simulink model "Model_10_1"  (R2021a)
settings: Solver=VariableStepAuto  StartTime=0.0  StopTime=10  RelTol=1e-3
InitFcn:
  | bx=25; %25
  | bl=50; %50
  | bc=0.1; %0.08
  | 
  | ml=2; %2
  | 
  | mc=0.5;
  | M2=0.5;
  | 
  | mt=5;
  | g=9.81;
  | l_ref=0.3; %0.3
  | l_ini=1;   %1
  | l=l_ini;
  | x_ref=1; %3
  | n1=1; %5
  | n2=1;
  | 
  | L_2=0;  %chieu dai day nang ha
  | 
  | theta1_ini=0*pi/180;
  | theta2_ini=0*pi/180;  %2*pi/180
  | 
  | L_tai=0.1;
  | %ADRC' s parameter caculation
  | %b0 = (1)/(mc+mt+ml);
  | b0=(ml+mc)/(mt*mc+2*ml*mc+mt*ml+ml^2+mc^2); %Enhanced-coupling
  | %k_ESO = 100;
  | k_ESO = 100;
  | T_set  = 3; %5;
  | 
  | s_cl = -5.85/T_set;
  | Kp   = s_cl^2;
  | Kd   = -2*s_cl;
  | 
  | s_ESO = k_ESO*s_cl;
  | l1        = -3*s_ESO;
  | l2        = 3*( s_ESO)^2;
  | l3        = -(s_ESO)^3;
  | 
  | %b1 = (mt+mc)/(mc*ml +mc*mt+ml*mt);
  | b1=1/(ml+mc);
  | k_ESO1 =100; %100
  | T_set1  = 3;   %3
  | s_cl1 = -5.85/T_set1;
  | Kp1   = s_cl1^2;
  | Kd1   = -2*s_cl1;
  | 
  | s_ESO1 = k_ESO1*s_cl1;
  | l11        = -3*s_ESO1;
  | l21        = 3*( s_ESO1)^2;
  | l31        = -(s_ESO1)^3;
  | 
  | 
  | %L1=l_ini;
  | L11=0.65;
  | L2=L_tai;
  | m1=2;
  | %m2=M2;
  | m=5;
  | ... (+35 lines)
libraries: neural x1372, simulink x44, simulink_extras x6
(part 44 of 58)

== matlab function Model_10_1/3_1_theta1 bang 0 n1=n2= 1/Ko co bx, bl, bc-1/Crane ==
  data: dx1 output; d1x input; l1 input; d1l1 input; the1 input; d1the1 input; the2 input; d1the2 input; Fx input; Fl input; dx2 output; dx3 output; dx4 output; dx5 output; dx6 output; m2 input; dx7 output; dx8 output; l2 input
function [dx1,dx2,dx3,dx4,dx5,dx6,dx7,dx8] = fcn(d1x,l1,d1l1,the1,d1the1,the2,d1the2,Fx,Fl,m2,l2)
 m =5; m1 =2; g =9.81;
 dx1=d1x;

 dx2 = (Fx*m2*cos(the1 - the2)^2 - Fx*m2 - Fx*m1 + Fx*m2*sin(the1 - the2)^2 + Fl*m1*sin(the1) + Fl*m2*sin(the1) - Fl*m2*sin(the1 - the2)*cos(the2) - d1the2^2*l2*m2^2*sin(the2) - g*m2^2*cos(the2)*sin(the2) - Fl*m2*cos(the1 - the2)^2*sin(the1) - g*m2^2*cos(the1 - the2)*sin(the1 - the2)*sin(the1)^2 + Fl*m2*cos(the1 - the2)*sin(the1 - the2)*cos(the1) + d1the2^2*l2*m2^2*cos(the1 - the2)*sin(the1) - d1the2^2*l2*m2^2*sin(the1 - the2)*cos(the1) - d1the2^2*l2*m1*m2*sin(the2) + g*m2^2*cos(the1 - the2)*cos(the1)*sin(the2) + g*m2^2*cos(the1 - the2)*cos(the2)*sin(the1) - g*m2^2*sin(the1 - the2)*cos(the1)*cos(the2) - g*m1*m2*cos(the2)*sin(the2) + g*m2^2*sin(the1 - the2)*sin(the1)*sin(the2) + d1the2^2*l2*m2^2*cos(the1 - the2)^2*sin(the2) - d1the2^2*l2*m2^2*cos(the1 - the2)^3*sin(the1) + d1the2^2*l2*m2^2*sin(the1 - the2)^3*cos(the1) - g*m2^2*cos(the1 - the2)^2*cos(the1)*sin(the1) + d1the2^2*l2*m2^2*sin(the1 - the2)^2*sin(the2) + g*m2^2*sin(the1 - the2)^2*cos(the1)*sin(the1) + g*m2^2*cos(the1 - the2)*sin(the1 - the2)*cos(the1)^2 - g*m1*m2*cos(the1 - the2)*sin(the1 - the2)*sin(the1)^2 + d1the2^2*l2*m1*m2*cos(the1 - the2)*sin(the1) - d1the2^2*l2*m1*m2*sin(the1 - the2)*cos(the1) + g*m1*m2*cos(the1 - the2)*cos(the1)*sin(the2) + g*m1*m2*cos(the1 - the2)*cos(the2)*sin(the1) - g*m1*m2*sin(the1 - the2)*cos(the1)*cos(the2) + g*m1*m2*sin(the1 - the2)*sin(the1)*sin(the2) + d1the2^2*l2*m2^2*cos(the1 - the2)^2*sin(the1 - the2)*cos(the1) - d1the2^2*l2*m2^2*cos(the1 - the2)*sin(the1 - the2)^2*sin(the1) - g*m1*m2*cos(the1 - the2)^2*cos(the1)*sin(the1) + g*m1*m2*sin(the1 - the2)^2*cos(the1)*sin(the1) + g*m1*m2*cos(the1 - the2)*sin(the1 - the2)*cos(the1)^2)/(m1^2*cos(the1)^2 - m*m2 - 2*m1*m2 - m*m1 + m2^2*cos(the1)^2 + m2^2*cos(the2)^2 + m1^2*sin(the1)^2 + m2^2*sin(the1)^2 + m2^2*cos(the1 - the2)^2 + m2^2*sin(the1 - the2)^2 - m1^2 - m2^2 + 2*m1*m2*cos(the1)^2 + m1*m2*cos(the2)^2 + 2*m1*m2*sin(the1)^2 + m*m2*cos(the1 - the2)^2 + m1*m2*cos(the1 - the2)^2 + m*m2*sin(the1 - the2)^2 + m1*m2*sin(the1 - the2)^2 - m2^2*cos(the1 - the2)^2*sin(the1)^2 - m2^2*sin(the1 - the2)^2*cos(the1)^2 - 2*m2^2*sin(the1 - the2)*cos(the2)*sin(the1) - 2*m2^2*cos(the1 - the2)*cos(the1)*cos(the2) - m1*m2*cos(the1 - the2)^2*sin(the1)^2 - m1*m2*sin(the1 - the2)^2*cos(the1)^2 + 2*m2^2*cos(the1 - the2)*sin(the1 - the2)*cos(the1)*sin(the1) - 2*m1*m2*sin(the1 - the2)*cos(the2)*sin(the1) - 2*m1*m2*cos(the1 - the2)*cos(the1)*cos(the2) + 2*m1*m2*cos(the1 - the2)*sin(the1 - the2)*cos(the1)*sin(the1));


 dx3=d1l1;

 dx4 = (Fx*m1^2*sin(the1) - Fl*m2^2 - Fl*m1^2 + Fx*m2^2*sin(the1) - d1the1^2*l1*m1^3 - d1the1^2*l1*m2^3 - g*m1^3*cos(the1) - g*m2^3*cos(the1) - Fl*m*m1 - Fl*m*m2 - 2*Fl*m1*m2 + Fl*m1^2*cos(the1)^2 + Fl*m2^2*cos(the1)^2 + Fl*m2^2*cos(the2)^2 + g*m1^3*cos(the1)^3 + g*m2^3*cos(the1)^3 + Fl*m2^2*cos(the1 - the2)^2 + 3*g*m1*m2^2*cos(the1)^3 + 3*g*m1^2*m2*cos(the1)^3 - Fx*m2^2*sin(the1 - the2)*cos(the2) - d1the2^2*l2*m2^3*cos(the1 - the2) + 2*Fx*m1*m2*sin(the1) + d1the1^2*l1*m1^3*cos(the1)^2 + d1the1^2*l1*m2^3*cos(the1)^2 + d1the1^2*l1*m2^3*cos(the2)^2 - g*m2^3*sin(the1 - the2)*sin(the2) + g*m2^3*cos(the1)*cos(the2)^2 + d1the1^2*l1*m1^3*sin(the1)^2 + d1the1^2*l1*m2^3*sin(the1)^2 + g*m1^3*cos(the1)*sin(the1)^2 + g*m2^3*cos(the1)*sin(the1)^2 + 2*Fl*m1*m2*cos(the1)^2 + Fl*m1*m2*cos(the2)^2 - Fx*m2^2*cos(the1 - the2)^2*sin(the1) + d1the1^2*l1*m2^3*cos(the1 - the2)^2 + d1the2^2*l2*m2^3*cos(the1 - the2)^3 - d1the1^2*l1*m*m1^2 - d1the1^2*l1*m*m2^2 - 3*d1the1^2*l1*m1*m2^2 - 3*d1the1^2*l1*m1^2*m2 + g*m2^3*cos(the1 - the2)^2*cos(the1) + d1the1^2*l1*m2^3*sin(the1 - the2)^2 - g*m*m1^2*cos(the1) - g*m*m2^2*cos(the1) - 3*g*m1*m2^2*cos(the1) - 3*g*m1^2*m2*cos(the1) + Fl*m*m2*cos(the1 - the2)^2 + Fl*m1*m2*cos(the1 - the2)^2 - g*m*m2^2*sin(the1 - the2)*sin(the2) - 2*g*m1*m2^2*sin(the1 - the2)*sin(the2) - g*m1^2*m2*sin(the1 - the2)*sin(the2) - d1the1^2*l1*m2^3*cos(the1 - the2)^2*sin(the1)^2 - d1the1^2*l1*m2^3*sin(the1 - the2)^2*cos(the1)^2 + 2*g*m1*m2^2*cos(the1)*cos(the2)^2 + g*m1^2*m2*cos(the1)*cos(the2)^2 + 3*d1the1^2*l1*m1*m2^2*sin(the1)^2 + 3*d1the1^2*l1*m1^2*m2*sin(the1)^2 + 3*g*m1*m2^2*cos(the1)*sin(the1)^2 + 3*g*m1^2*m2*cos(the1)*sin(the1)^2 + d1the2^2*l2*m2^3*sin(the1)*sin(the2) - 2*Fl*m2^2*cos(the1 - the2)*cos(the1)*cos(the2) + d1the1^2*l1*m*m2^2*cos(the1 - the2)^2 + 2*d1the1^2*l1*m1*m2^2*cos(the1 - the2)^2 + d1the1^2*l1*m1^2*m2*cos(the1 - the2)^2 + d1the2^2*l2*m*m2^2*cos(the1 - the2)^3 + d1the2^2*l2*m1*m2^2*cos(the1 - the2)^3 + g*m2^3*cos(the2)*sin(the1)*sin(the2) + g*m*m2^2*cos(the1 - the2)^2*cos(the1) + 2*g*m1*m2^2*cos(the1 - the2)^2*cos(the1) + g*m1^2*m2*cos(the1 - the2)^2*cos(the1) + d1the1^2*l1*m*m2^2*sin(the1 - the2)^2 + 2*d1the1^2*l1*m1*m2^2*sin(the1 - the2)^2 + d1the1^2*l1*m1^2*m2*sin(the1 - the2)^2 + Fx*m2^2*cos(the1 - the2)*sin(the1 - the2)*cos(the1) - Fx*m1*m2*sin(the1 - the2)*cos(the2) + d1the2^2*l2*m2^3*cos(the1 - the2)*cos(the1)^2 + d1the2^2*l2*m2^3*cos(the1 - the2)*cos(the2)^2 + g*m2^3*cos(the1 - the2)*sin(the1 - the2)*sin(the1) - 2*g*m2^3*cos(the1 - the2)*cos(the1)^2*cos(the2) - g*m2^3*cos(the1 - the2)*cos(the2)*sin(the1)^2 + g*m2^3*sin(the1 - the2)*cos(the1)^2*sin(the2) - Fx*m1*m2*cos(the1 - the2)^2*sin(the1) - d1the2^2*l2*m*m2^2*cos(the1 - the2) - 2*d1the2^2*l2*m1*m2^2*cos(the1 - the2) - d1the2^2*l2*m1^2*m2*cos(the1 - the2) - 2*d1the1^2*l1*m*m1*m2 + d1the2^2*l2*m2^3*cos(the1 - the2)*sin(the1 - the2)^2 - 2*g*m*m1*m2*cos(the1) + 3*d1the1^2*l1*m1*m2^2*cos(the1)^2 + 3*d1the1^2*l1*m1^2*m2*cos(the1)^2 + 2*d1the1^2*l1*m1*m2^2*cos(the2)^2 + d1the1^2*l1*m1^2*m2*cos(the2)^2 + 2*d1the2^2*l2*m1*m2^2*cos(the1 - the2)*cos(the1)^2 + d1the2^2*l2*m1^2*m2*cos(the1 - the2)*cos(the1)^2 + d1the2^2*l2*m1*m2^2*cos(the1 - the2)*cos(the2)^2 + g*m*m2^2*cos(the1 - the2)*sin(the1 - the2)*sin(the1) + 2*g*m1*m2^2*cos(the1 - the2)*sin(the1 - the2)*sin(the1) + g*m1^2*m2*cos(the1 - the2)*sin(the1 - the2)*sin(the1) - g*m*m1*m2*sin(the1 - the2)*sin(the2) - 2*d1the1^2*l1*m2^3*cos(the1 - the2)*cos(the1)*cos(the2) - 4*g*m1*m2^2*cos(the1 - the2)*cos(the1)^2*cos(the2) - 2*g*m1^2*m2*cos(the1 - the2)*cos(the1)^2*cos(the2) - 2*g*m1*m2^2*cos(the1 - the2)*cos(the2)*sin(the1)^2 - g*m1^2*m2*cos(the1 - the2)*cos(the2)*sin(the1)^2 - 2*d1the1^2*l1*m2^3*sin(the1 - the2)*cos(the2)*sin(the1) + d1the2^2*l2*m2^3*sin(the1 - the2)*cos(the1)*sin(the1) - d1the2^2*l2*m2^3*sin(the1 - the2)*cos(the2)*sin(the2) + 2*g*m1*m2^2*sin(the1 - the2)*cos(the1)^2*sin(the2) + g*m1^2*m2*sin(the1 - the2)*cos(the1)^2*sin(the2) - 2*Fl*m1*m2*cos(the1 - the2)*cos(the1)*cos(the2) + d1the1^2*l1*m*m1*m2*cos(the1 - the2)^2 - g*m2^3*cos(the1 - the2)*cos(the1)*sin(the1)*sin(the2) - g*m2^3*sin(the1 - the2)*cos(the1)*cos(the2)*sin(the1) + d1the2^2*l2*m*m2^2*cos(the1 - the2)*sin(the1 - the2)^2 + d1the2^2*l2*m1*m2^2*cos(the1 - the2)*sin(the1 - the2)^2 + g*m*m1*m2*cos(the1 - the2)^2*cos(the1) + d1the1^2*l1*m*m1*m2*sin(the1 - the2)^2 - 2*d1the2^2*l2*m2^3*cos(the1 - the2)^2*cos(the1)*cos(the2) - 2*d1the1^2*l1*m1*m2^2*cos(the1 - the2)^2*sin(the1)^2 - 2*d1the1^2*l1*m1*m2^2*sin(the1 - the2)^2*cos(the1)^2 - d1the1^2*l1*m1^2*m2*cos(the1 - the2)^2*sin(the1)^2 - d1the1^2*l1*m1^2*m2*sin(the1 - the2)^2*cos(the1)^2 + Fx*m1*m2*cos(the1 - the2)*sin(the1 - the2)*cos(the1) - d1the2^2*l2*m2^3*sin(the1 - the2)^2*cos(the1)*cos(the2) - d1the2^2*l2*m2^3*cos(the1 - the2)^2*sin(the1)*sin(the2) + 2*d1the2^2*l2*m1*m2^2*sin(the1)*sin(the2) + d1the2^2*l2*m1^2*m2*sin(the1)*sin(the2) + 2*g*m1*m2^2*cos(the2)*sin(the1)*sin(the2) + g*m1^2*m2*cos(the2)*sin(the1)*sin(the2) - d1the2^2*l2*m*m1*m2*cos(the1 - the2) - d1the2^2*l2*m1*m2^2*cos(the1 - the2)^2*sin(the1)*sin(the2) + g*m*m1*m2*cos(the1 - the2)*sin(the1 - the2)*sin(the1) + 2*d1the1^2*l1*m2^3*cos(the1 - the2)*sin(the1 - the2)*cos(the1)*sin(the1) + d1the2^2*l2*m2^3*cos(the1 - the2)*sin(the1 - the2)*cos(the1)*sin(the2) - d1the2^2*l2*m2^3*cos(the1 - the2)*sin(the1 - the2)*cos(the2)*sin(the1) - 4*d1the1^2*l1*m1*m2^2*cos(the1 - the2)*cos(the1)*cos(the2) - 2*d1the1^2*l1*m1^2*m2*cos(the1 - the2)*cos(the1)*cos(the2) - 4*d1the1^2*l1*m1*m2^2*sin(the1 - the2)*cos(the2)*sin(the1) - 2*d1the1^2*l1*m1^2*m2*sin(the1 - the2)*cos(the2)*sin(the1) + 2*d1the2^2*l2*m1*m2^2*sin(the1 - the2)*cos(the1)*sin(the1) + d1the2^2*l2*m1^2*m2*sin(the1 - the2)*cos(the1)*sin(the1) - d1the2^2*l2*m1*m2^2*sin(the1 - the2)*cos(the2)*sin(the2) - 2*g*m1*m2^2*cos(the1 - the2)*cos(the1)*sin(the1)*sin(the2) - 2*g*m1*m2^2*sin(the1 - the2)*cos(the1)*cos(the2)*sin(the1) - g*m1^2*m2*cos(the1 - the2)*cos(the1)*sin(the1)*sin(the2) - g*m1^2*m2*sin(the1 - the2)*cos(the1)*cos(the2)*sin(the1) - 2*d1the2^2*l2*m1*m2^2*cos(the1 - the2)^2*cos(the1)*cos(the2) - d1the2^2*l2*m1*m2^2*sin(the1 - the2)^2*cos(the1)*cos(the2) + 4*d1the1^2*l1*m1*m2^2*cos(the1 - the2)*sin(the1 - the2)*cos(the1)*sin(the1) + 2*d1the1^2*l1*m1^2*m2*cos(the1 - the2)*sin(the1 - the2)*cos(the1)*sin(the1) + d1the2^2*l2*m1*m2^2*cos(the1 - the2)*sin(the1 - the2)*cos(the1)*sin(the2) - d1the2^2*l2*m1*m2^2*cos(the1 - the2)*sin(the1 - the2)*cos(the2)*sin(the1))/((m1 + m2)*(m1^2*cos(the1)^2 - m*m2 - 2*m1*m2 - m*m1 + m2^2*cos(the1)^2 + m2^2*cos(the2)^2 + m1^2*sin(the1)^2 + m2^2*sin(the1)^2 + m2^2*cos(the1 - the2)^2 + m2^2*sin(the1 - the2)^2 - m1^2 - m2^2 + 2*m1*m2*cos(the1)^2 + m1*m2*cos(the2)^2 + 2*m1*m2*sin(the1)^2 + m*m2*cos(the1 - the2)^2 + m1*m2*cos(the1 - the2)^2 + m*m2*sin(the1 - the2)^2 + m1*m2*sin(the1 - the2)^2 - m2^2*cos(the1 - the2)^2*sin(the1)^2 - m2^2*sin(the1 - the2)^2*cos(the1)^2 - 2*m2^2*sin(the1 - the2)*cos(the2)*sin(the1) - 2*m2^2*cos(the1 - the2)*cos(the1)*cos(the2) - m1*m2*cos(the1 - the2)^2*sin(the1)^2 - m1*m2*sin(the1 - the2)^2*cos(the1)^2 + 2*m2^2*cos(the1 - the2)*sin(the1 - the2)*cos(the1)*sin(the1) - 2*m1*m2*sin(the1 - the2)*cos(the2)*sin(the1) - 2*m1*m2*cos(the1 - the2)*cos(the1)*cos(the2) + 2*m1*m2*cos(the1 - the2)*sin(the1 - the2)*cos(the1)*sin(the1)));


 dx5=d1the1;

 dx6 = -(g*m1^3*sin(the1)^3 - Fx*m2^2*cos(the1) - g*m1^3*sin(the1) - g*m2^3*sin(the1) - Fx*m1^2*cos(the1) + g*m2^3*sin(the1)^3 - 2*d1l1*d1the1*m1^3 - 2*d1l1*d1the1*m2^3 + 2*d1l1*d1the1*m1^3*cos(the1)^2 + 2*d1l1*d1the1*m2^3*cos(the1)^2 + 2*d1l1*d1the1*m2^3*cos(the2)^2 + Fl*m1^2*cos(the1)*sin(the1) + Fl*m2^2*cos(the1)*sin(the1) + 2*d1l1*d1the1*m1^3*sin(the1)^2 + 2*d1l1*d1the1*m2^3*sin(the1)^2 + 3*g*m1*m2^2*sin(the1)^3 + 3*g*m1^2*m2*sin(the1)^3 + Fx*m2^2*cos(the1 - the2)*cos(the2) - 2*Fx*m1*m2*cos(the1) + 2*d1l1*d1the1*m2^3*cos(the1 - the2)^2 - 2*d1l1*d1the1*m*m1^2 - 2*d1l1*d1the1*m*m2^2 - 6*d1l1*d1the1*m1*m2^2 - 6*d1l1*d1the1*m1^2*m2 + 2*d1l1*d1the1*m2^3*sin(the1 - the2)^2 - d1the2^2*l2*m2^3*sin(the1 - the2) + g*m2^3*cos(the1 - the2)*sin(the2) + Fl*m2^2*cos(the1 - the2)*sin(the1 - the2) + g*m1^3*cos(the1)^2*sin(the1) + g*m2^3*cos(the1)^2*sin(the1) + g*m2^3*cos(the2)^2*sin(the1) + Fx*m2^2*sin(the1 - the2)^2*cos(the1) + d1the2^2*l2*m2^3*sin(the1 - the2)^3 - g*m*m1^2*sin(the1) - g*m*m2^2*sin(the1) - 3*g*m1*m2^2*sin(the1) - 3*g*m1^2*m2*sin(the1) + g*m2^3*sin(the1 - the2)^2*sin(the1) - d1the2^2*l2*m2^3*cos(the1)*sin(the2) + 3*g*m1*m2^2*cos(the1)^2*sin(the1) + 3*g*m1^2*m2*cos(the1)^2*sin(the1) + 2*g*m1*m2^2*cos(the2)^2*sin(the1) + g*m1^2*m2*cos(the2)^2*sin(the1) - g*m2^3*cos(the1)*cos(the2)*sin(the2) - Fl*m2^2*cos(the1 - the2)*cos(the2)*sin(the1) - Fl*m2^2*sin(the1 - the2)*cos(the1)*cos(the2) + 2*Fl*m1*m2*cos(the1)*sin(the1) + d1the2^2*l2*m*m2^2*sin(the1 - the2)^3 + d1the2^2*l2*m1*m2^2*sin(the1 - the2)^3 + g*m*m2^2*sin(the1 - the2)^2*sin(the1) + 2*g*m1*m2^2*sin(the1 - the2)^2*sin(the1) + g*m1^2*m2*sin(the1 - the2)^2*sin(the1) + Fx*m1*m2*cos(the1 - the2)*cos(the2) - 4*d1l1*d1the1*m*m1*m2 - Fx*m2^2*cos(the1 - the2)*sin(the1 - the2)*sin(the1) + g*m2^3*cos(the1 - the2)*sin(the1 - the2)*cos(the1) + 6*d1l1*d1the1*m1*m2^2*cos(the1)^2 + 6*d1l1*d1the1*m1^2*m2*cos(the1)^2 + 4*d1l1*d1the1*m1*m2^2*cos(the2)^2 + 2*d1l1*d1the1*m1^2*m2*cos(the2)^2 - 2*d1l1*d1the1*m2^3*cos(the1 - the2)^2*sin(the1)^2 - 2*d1l1*d1the1*m2^3*sin(the1 - the2)^2*cos(the1)^2 + Fl*m*m2*cos(the1 - the2)*sin(the1 - the2) + Fl*m1*m2*cos(the1 - the2)*sin(the1 - the2) + 6*d1l1*d1the1*m1*m2^2*sin(the1)^2 + 6*d1l1*d1the1*m1^2*m2*sin(the1)^2 + d1the2^2*l2*m2^3*sin(the1 - the2)*cos(the2)^2 - g*m2^3*sin(the1 - the2)*cos(the1)^2*cos(the2) + d1the2^2*l2*m2^3*sin(the1 - the2)*sin(the1)^2 + 2*d1l1*d1the1*m*m2^2*cos(the1 - the2)^2 + 4*d1l1*d1the1*m1*m2^2*cos(the1 - the2)^2 + 2*d1l1*d1the1*m1^2*m2*cos(the1 - the2)^2 - g*m2^3*cos(the1 - the2)*sin(the1)^2*sin(the2) - 2*g*m2^3*sin(the1 - the2)*cos(the2)*sin(the1)^2 + Fx*m1*m2*sin(the1 - the2)^2*cos(the1) + 2*d1l1*d1the1*m*m2^2*sin(the1 - the2)^2 + 4*d1l1*d1the1*m1*m2^2*sin(the1 - the2)^2 + 2*d1l1*d1the1*m1^2*m2*sin(the1 - the2)^2 + d1the2^2*l2*m2^3*cos(the1 - the2)^2*sin(the1 - the2) - d1the2^2*l2*m*m2^2*sin(the1 - the2) - 2*d1the2^2*l2*m1*m2^2*sin(the1 - the2) - d1the2^2*l2*m1^2*m2*sin(the1 - the2) + g*m*m2^2*cos(the1 - the2)*sin(the2) + 2*g*m1*m2^2*cos(the1 - the2)*sin(the2) + g*m1^2*m2*cos(the1 - the2)*sin(the2) - 2*g*m*m1*m2*sin(the1) + g*m*m1*m2*cos(the1 - the2)*sin(the2) - 4*d1l1*d1the1*m1*m2^2*cos(the1 - the2)^2*sin(the1)^2 - 4*d1l1*d1the1*m1*m2^2*sin(the1 - the2)^2*cos(the1)^2 - 2*d1l1*d1the1*m1^2*m2*cos(the1 - the2)^2*sin(the1)^2 - 2*d1l1*d1the1*m1^2*m2*sin(the1 - the2)^2*cos(the1)^2 + d1the2^2*l2*m1*m2^2*sin(the1 - the2)*cos(the2)^2 + d1the2^2*l2*m2^3*cos(the1 - the2)*cos(the1)*sin(the1) + d1the2^2*l2*m2^3*cos(the1 - the2)*cos(the2)*sin(the2) - 2*g*m1*m2^2*sin(the1 - the2)*cos(the1)^2*cos(the2) - g*m1^2*m2*sin(the1 - the2)*cos(the1)^2*cos(the2) + 2*d1the2^2*l2*m1*m2^2*sin(the1 - the2)*sin(the1)^2 + d1the2^2*l2*m1^2*m2*sin(the1 - the2)*sin(the1)^2 - g*m2^3*cos(the1 - the2)*cos(the1)*cos(the2)*sin(the1) - 2*g*m1*m2^2*cos(the1 - the2)*sin(the1)^2*sin(the2) - 4*g*m1*m2^2*sin(the1 - the2)*cos(the2)*sin(the1)^2 - g*m1^2*m2*cos(the1 - the2)*sin(the1)^2*sin(the2) - 2*g*m1^2*m2*sin(the1 - the2)*cos(the2)*sin(the1)^2 - Fl*m1*m2*cos(the1 - the2)*cos(the2)*sin(the1) - Fl*m1*m2*sin(the1 - the2)*cos(the1)*cos(the2) + d1the2^2*l2*m*m2^2*cos(the1 - the2)^2*sin(the1 - the2) + d1the2^2*l2*m1*m2^2*cos(the1 - the2)^2*sin(the1 - the2) + g*m2^3*sin(the1 - the2)*cos(the1)*sin(the1)*sin(the2) + g*m*m1*m2*sin(the1 - the2)^2*sin(the1) - d1the2^2*l2*m2^3*cos(the1 - the2)^2*cos(the2)*sin(the1) - 2*d1the2^2*l2*m1*m2^2*cos(the1)*sin(the2) - d1the2^2*l2*m1^2*m2*cos(the1)*sin(the2) - Fx*m1*m2*cos(the1 - the2)*sin(the1 - the2)*sin(the1) + d1the2^2*l2*m2^3*sin(the1 - the2)^2*cos(the1)*sin(the2) - 2*d1the2^2*l2*m2^3*sin(the1 - the2)^2*cos(the2)*sin(the1) - 2*g*m1*m2^2*cos(the1)*cos(the2)*sin(the2) - g*m1^2*m2*cos(the1)*cos(the2)*sin(the2) - 4*d1l1*d1the1*m2^3*cos(the1 - the2)*cos(the1)*cos(the2) - 4*d1l1*d1the1*m2^3*sin(the1 - the2)*cos(the2)*sin(the1) + 2*d1l1*d1the1*m*m1*m2*cos(the1 - the2)^2 + 2*d1l1*d1the1*m*m1*m2*sin(the1 - the2)^2 - d1the2^2*l2*m*m1*m2*sin(the1 - the2) + g*m*m2^2*cos(the1 - the2)*sin(the1 - the2)*cos(the1) + 2*g*m1*m2^2*cos(the1 - the2)*sin(the1 - the2)*cos(the1) + g*m1^2*m2*cos(the1 - the2)*sin(the1 - the2)*cos(the1) + d1the2^2*l2*m1*m2^2*sin(the1 - the2)^2*cos(the1)*sin(the2) - 2*d1the2^2*l2*m1*m2^2*sin(the1 - the2)^2*cos(the2)*sin(the1) + g*m*m1*m2*cos(the1 - the2)*sin(the1 - the2)*cos(the1) - 8*d1l1*d1the1*m1*m2^2*cos(the1 - the2)*cos(the1)*cos(the2) - 4*d1l1*d1the1*m1^2*m2*cos(the1 - the2)*cos(the1)*cos(the2) - d1the2^2*l2*m2^3*cos(the1 - the2)*sin(the1 - the2)*cos(the1)*cos(the2) - 8*d1l1*d1the1*m1*m2^2*sin(the1 - the2)*cos(the2)*sin(the1) - 4*d1l1*d1the1*m1^2*m2*sin(the1 - the2)*cos(the2)*sin(the1) - d1the2^2*l2*m2^3*cos(the1 - the2)*sin(the1 - the2)*sin(the1)*sin(the2) + 2*d1the2^2*l2*m1*m2^2*cos(the1 - the2)*cos(the1)*sin(the1) + d1the2^2*l2*m1^2*m2*cos(the1 - the2)*cos(the1)*sin(the1) + d1the2^2*l2*m1*m2^2*cos(the1 - the2)*cos(the2)*sin(the2) - 2*g*m1*m2^2*cos(the1 - the2)*cos(the1)*cos(the2)*sin(the1) - g*m1^2*m2*cos(the1 - the2)*cos(the1)*cos(the2)*sin(the1) + 2*g*m1*m2^2*sin(the1 - the2)*cos(the1)*sin(the1)*sin(the2) + g*m1^2*m2*sin(the1 - the2)*cos(the1)*sin(the1)*sin(the2) + 4*d1l1*d1the1*m2^3*cos(the1 - the2)*sin(the1 - the2)*cos(the1)*sin(the1) - d1the2^2*l2*m1*m2^2*cos(the1 - the2)^2*cos(the2)*sin(the1) + 8*d1l1*d1the1*m1*m2^2*cos(the1 - the2)*sin(the1 - the2)*cos(the1)*sin(the1) + 4*d1l1*d1the1*m1^2*m2*cos(the1 - the2)*sin(the1 - the2)*cos(the1)*sin(the1) - d1the2^2*l2*m1*m2^2*cos(the1 - the2)*sin(the1 - the2)*cos(the1)*cos(the2) - d1the2^2*l2*m1*m2^2*cos(the1 - the2)*sin(the1 - the2)*sin(the1)*sin(the2))/(l1*(m1 + m2)*(m1^2*cos(the1)^2 - m*m2 - 2*m1*m2 - m*m1 + m2^2*cos(the1)^2 + m2^2*cos(the2)^2 + m1^2*sin(the1)^2 + m2^2*sin(the1)^2 + m2^2*cos(the1 - the2)^2 + m2^2*sin(the1 - the2)^2 - m1^2 - m2^2 + 2*m1*m2*cos(the1)^2 + m1*m2*cos(the2)^2 + 2*m1*m2*sin(the1)^2 + m*m2*cos(the1 - the2)^2 + m1*m2*cos(the1 - the2)^2 + m*m2*sin(the1 - the2)^2 + m1*m2*sin(the1 - the2)^2 - m2^2*cos(the1 - the2)^2*sin(the1)^2 - m2^2*sin(the1 - the2)^2*cos(the1)^2 - 2*m2^2*sin(the1 - the2)*cos(the2)*sin(the1) - 2*m2^2*cos(the1 - the2)*cos(the1)*cos(the2) - m1*m2*cos(the1 - the2)^2*sin(the1)^2 - m1*m2*sin(the1 - the2)^2*cos(the1)^2 + 2*m2^2*cos(the1 - the2)*sin(the1 - the2)*cos(the1)*sin(the1) - 2*m1*m2*sin(the1 - the2)*cos(the2)*sin(the1) - 2*m1*m2*cos(the1 - the2)*cos(the1)*cos(the2) + 2*m1*m2*cos(the1 - the2)*sin(the1 - the2)*cos(the1)*sin(the1)));

 dx7=d1the2;

 dx8 = -(Fx*m1*sin(the1 - the2)*sin(the1) - Fl*m1*sin(the1 - the2) - Fl*m2*sin(the1 - the2) - g*m1^2*sin(the2) - g*m2^2*sin(the2) - Fx*m1*cos(the2) - Fx*m2*cos(the2) - Fl*m*sin(the1 - the2) + Fx*m2*sin(the1 - the2)*sin(the1) + Fl*m1*sin(the1 - the2)*cos(the1)^2 + Fl*m2*sin(the1 - the2)*cos(the1)^2 + g*m1^2*cos(the1 - the2)*sin(the1) - g*m1^2*sin(the1 - the2)*cos(the1) + g*m2^2*cos(the1 - the2)*sin(the1) - g*m2^2*sin(the1 - the2)*cos(the1) - g*m*m1*sin(the2) - g*m*m2*sin(the2) - 2*g*m1*m2*sin(the2) + g*m1^2*cos(the1)^2*sin(the2) + g*m2^2*cos(the1)^2*sin(the2) + g*m1^2*sin(the1)^2*sin(the2) + g*m2^2*sin(the1)^2*sin(the2) + Fl*m1*cos(the2)*sin(the1) + Fl*m2*cos(the2)*sin(the1) - g*m1^2*cos(the1 - the2)*sin(the1)^3 + g*m1^2*sin(the1 - the2)*cos(the1)^3 - g*m2^2*cos(the1 - the2)*sin(the1)^3 + g*m2^2*sin(the1 - the2)*cos(the1)^3 + Fx*m1*cos(the1 - the2)*cos(the1) + Fx*m2*cos(the1 - the2)*cos(the1) - d1the2^2*l2*m2^2*cos(the2)*sin(the2) + g*m*m1*cos(the1 - the2)*sin(the1) - g*m*m1*sin(the1 - the2)*cos(the1) + g*m*m2*cos(the1 - the2)*sin(the1) - g*m*m2*sin(the1 - the2)*cos(the1) + 2*g*m1*m2*cos(the1 - the2)*sin(the1) - 2*g*m1*m2*sin(the1 - the2)*cos(the1) - g*m1^2*cos(the1 - the2)*cos(the1)^2*sin(the1) - g*m2^2*cos(the1 - the2)*cos(the1)^2*sin(the1) + 2*g*m1*m2*cos(the1)^2*sin(the2) + g*m1^2*sin(the1 - the2)*cos(the1)*sin(the1)^2 + g*m2^2*sin(the1 - the2)*cos(the1)*sin(the1)^2 + 2*g*m1*m2*sin(the1)^2*sin(the2) - Fl*m1*cos(the1 - the2)*cos(the1)*sin(the1) - Fl*m2*cos(the1 - the2)*cos(the1)*sin(the1) - 2*g*m1*m2*cos(the1 - the2)*sin(the1)^3 + 2*g*m1*m2*sin(the1 - the2)*cos(the1)^3 + d1the2^2*l2*m2^2*cos(the1 - the2)*cos(the1)*sin(the2) + d1the2^2*l2*m2^2*cos(the1 - the2)*cos(the2)*sin(the1) - d1the2^2*l2*m2^2*sin(the1 - the2)*cos(the1)*cos(the2) - d1the2^2*l2*m1*m2*cos(the2)*sin(the2) + d1the2^2*l2*m2^2*sin(the1 - the2)*sin(the1)*sin(the2) - d1the2^2*l2*m2^2*cos(the1 - the2)^2*cos(the1)*sin(the1) + d1the2^2*l2*m2^2*sin(the1 - the2)^2*cos(the1)*sin(the1) + d1the2^2*l2*m2^2*cos(the1 - the2)*sin(the1 - the2)*cos(the1)^2 - d1the2^2*l2*m2^2*cos(the1 - the2)*sin(the1 - the2)*sin(the1)^2 - 2*g*m1*m2*cos(the1 - the2)*cos(the1)^2*sin(the1) + 2*g*m1*m2*sin(the1 - the2)*cos(the1)*sin(the1)^2 + d1the2^2*l2*m1*m2*cos(the1 - the2)*cos(the1)*sin(the2) + d1the2^2*l2*m1*m2*cos(the1 - the2)*cos(the2)*sin(the1) - d1the2^2*l2*m1*m2*sin(the1 - the2)*cos(the1)*cos(the2) + d1the2^2*l2*m1*m2*sin(the1 - the2)*sin(the1)*sin(the2) - d1the2^2*l2*m1*m2*cos(the1 - the2)^2*cos(the1)*sin(the1) + d1the2^2*l2*m1*m2*sin(the1 - the2)^2*cos(the1)*sin(the1) + d1the2^2*l2*m1*m2*cos(the1 - the2)*sin(the1 - the2)*cos(the1)^2 - d1the2^2*l2*m1*m2*cos(the1 - the2)*sin(the1 - the2)*sin(the1)^2)/(l2*(m1^2*cos(the1)^2 - m*m2 - 2*m1*m2 - m*m1 + m2^2*cos(the1)^2 + m2^2*cos(the2)^2 + m1^2*sin(the1)^2 + m2^2*sin(the1)^2 + m2^2*cos(the1 - the2)^2 + m2^2*sin(the1 - the2)^2 - m1^2 - m2^2 + 2*m1*m2*cos(the1)^2 + m1*m2*cos(the2)^2 + 2*m1*m2*sin(the1)^2 + m*m2*cos(the1 - the2)^2 + m1*m2*cos(the1 - the2)^2 + m*m2*sin(the1 - the2)^2 + m1*m2*sin(the1 - the2)^2 - m2^2*cos(the1 - the2)^2*sin(the1)^2 - m2^2*sin(the1 - the2)^2*cos(the1)^2 - 2*m2^2*sin(the1 - the2)*cos(the2)*sin(the1) - 2*m2^2*cos(the1 - the2)*cos(the1)*cos(the2) - m1*m2*cos(the1 - the2)^2*sin(the1)^2 - m1*m2*sin(the1 - the2)^2*cos(the1)^2 + 2*m2^2*cos(the1 - the2)*sin(the1 - the2)*cos(the1)*sin(the1) - 2*m1*m2*sin(the1 - the2)*cos(the2)*sin(the1) - 2*m1*m2*cos(the1 - the2)*cos(the1)*cos(the2) + 2*m1*m2*cos(the1 - the2)*sin(the1 - the2)*cos(the1)*sin(the1)));
